simulink model "passive_balance"  (R2023b)
settings: Solver=VariableStepAuto  StartTime=0.0  StopTime=inf  RelTol=1e-3
undefined symbols (not defined in the file): Ion, LF, Lithium
libraries: instrumentseriallib x9, spsSeriesRLCBranchLib x4, spsBatteryLib x3, spsIGBTLib x3, etargetslib x3, spsIdealSwitchLib x2, spsDCVoltageSourceLib x1, spspowerguiLib x1
settings Model: Creator=ASUS  LastModifiedBy=Bramantio

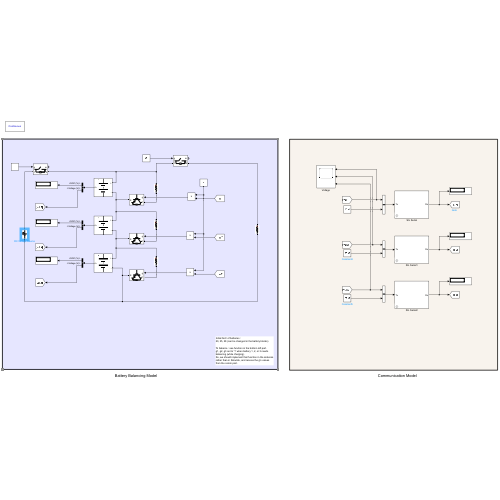
[thumbnail: Simulink's stored preview of the top-level diagram]
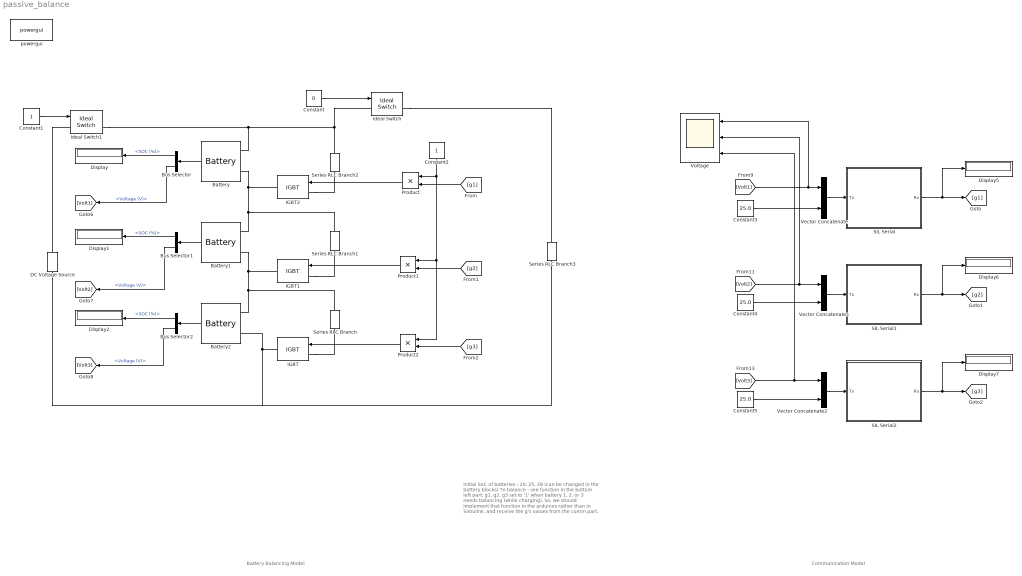
== system passive_balance ==
  note: Initial SoC of batteries :
      | 20, 25, 28 (can be changed in the battery blocks)
      |
      | To balance : see function in the bottom left part.
      | g1, g2, g3 set to '1' when battery 1, 2, or 3 needs
      | balancing (while charging).
      | So, we should implement that function in the arduinos
      | rather than in Simulink, and receive the g's values
      | from the comm part.
  note: Battery Balancing Model
  note: Communication Model
  Battery : spsBatteryLib/Battery  BatType=Lithium-Ion  ShowTempParam=off  ThermalPreset=no  ShowAgeParam=off  NomV=3.2  NomQ=180  SOC=20  Batt_Tr=30  PresetModel=on  MaxQ=180  MinV=2.4  FullV=3.7248  Dis_rate=78.2609  R=0.00017778  Normal_OP=162.7826  expZone="[3.4572      8.8435]"  current=[6.5 13 32.5]  Units=Time  Tci=20  NomT=20  T2=-30  MaxQ2=4.8  FullV2=7.1  Normal_OP2=5.655  expZone2="[6.58           1]"  Rca=0.6  ti=2000  Dp=0  Neq0=0  Tsim=1e6  Ta1=25  Qeol=5.4*0.9  Reol=0.013333*1.2  Char_age=[2.3478, 3]  Dis_age=[2.3478, 10]  N1=1500  N2=10500  N3=1000  N4=1400  Ta2=45  N5=950
  Battery1 : spsBatteryLib/Battery  BatType=Lithium-Ion  ShowTempParam=off  ThermalPreset=no  ShowAgeParam=off  NomV=3.2  NomQ=180  SOC=25  Batt_Tr=30  PresetModel=on  MaxQ=180  MinV=2.4  FullV=3.7248  Dis_rate=78.2609  R=0.00017778  Normal_OP=162.7826  expZone="[3.4572      8.8435]"  current=[6.5 13 32.5]  Units=Time  Tci=20  NomT=20  T2=-30  MaxQ2=4.8  FullV2=7.1  Normal_OP2=5.655  expZone2="[6.58           1]"  Rca=0.6  ti=2000  Dp=0  Neq0=0  Tsim=1e6  Ta1=25  Qeol=5.4*0.9  Reol=0.013333*1.2  Char_age=[2.3478, 3]  Dis_age=[2.3478, 10]  N1=1500  N2=10500  N3=1000  N4=1400  Ta2=45  N5=950
  Battery2 : spsBatteryLib/Battery  BatType=Lithium-Ion  ShowTempParam=off  ThermalPreset=no  ShowAgeParam=off  NomV=3.2  NomQ=180  SOC=28  Batt_Tr=30  PresetModel=on  MaxQ=180  MinV=2.4  FullV=3.7248  Dis_rate=78.2609  R=0.00017778  Normal_OP=162.7826  expZone="[3.4572      8.8435]"  current=[6.5 13 32.5]  Units=Time  Tci=20  NomT=20  T2=-30  MaxQ2=4.8  FullV2=7.1  Normal_OP2=5.655  expZone2="[6.58           1]"  Rca=0.6  ti=2000  Dp=0  Neq0=0  Tsim=1e6  Ta1=25  Qeol=5.4*0.9  Reol=0.013333*1.2  Char_age=[2.3478, 3]  Dis_age=[2.3478, 10]  N1=1500  N2=10500  N3=1000  N4=1400  Ta2=45  N5=950
  Bus Selector : BusSelector  OutputSignals=SOC (%),Voltage (V)
  Bus Selector1 : BusSelector  OutputSignals=SOC (%),Voltage (V)
  Bus Selector2 : BusSelector  OutputSignals=SOC (%),Voltage (V)
  Constant : Constant  Value=0
  Constant1 : Constant
  Constant2 : Constant
  Constant3 : Constant  Value=25.0
  Constant4 : Constant  Value=25.0
  Constant5 : Constant  Value=25.0
  DC Voltage Source : spsDCVoltageSourceLib/DC Voltage Source  Amplitude=10  Measurements=None
  Display{,1..2,5..7} (6 alike) : Display
  IGBT : spsIGBTLib/IGBT  Ron=0.001  Lon=0  Vf=1  Tf=1e-6  Tt=2e-6  IC=0  Rs=1e5  Cs=inf  Measurements=off
  IGBT1 : spsIGBTLib/IGBT  Ron=0.001  Lon=0  Vf=1  Tf=1e-6  Tt=2e-6  IC=0  Rs=1e5  Cs=inf  Measurements=off
  IGBT2 : spsIGBTLib/IGBT  Ron=0.001  Lon=0  Vf=1  Tf=1e-6  Tt=2e-6  IC=0  Rs=1e5  Cs=inf  Measurements=off
  Ideal Switch : spsIdealSwitchLib/Ideal Switch  Ron=0.001  Lon=0  IC=0  Rs=1e5  Cs=inf  Measurements=on
  Ideal Switch1 : spsIdealSwitchLib/Ideal Switch  Ron=0.001  Lon=0  IC=0  Rs=1e5  Cs=inf  Measurements=on
  Product : Product
  Product1 : Product
  Product2 : Product
  SIL Serial : Subsystem  mask{comport=COM3, data_size=1, sample_time=0.5, baud_rate=115200}
      mask prompts: comport "Serial Port (ex. "COM3")"; data_size "Data Size"; sample_time "Sample Time"; baud_rate "Baud Rate"
  SIL Serial1 : Subsystem  mask{comport=COM7, data_size=1, sample_time=0.5, baud_rate=115200}
      mask prompts: comport "Serial Port (ex. "COM3")"; data_size "Data Size"; sample_time "Sample Time"; baud_rate "Baud Rate"
  SIL Serial2 : Subsystem  mask{comport=COM8, data_size=1, sample_time=0.5, baud_rate=115200}
      mask prompts: comport "Serial Port (ex. "COM3")"; data_size "Data Size"; sample_time "Sample Time"; baud_rate "Baud Rate"
  Series RLC Branch{,1..3} (4 alike) : spsSeriesRLCBranchLib/Series RLC Branch  LConnTagsString=__new0  RConnTagsString=__new0  BranchType=R  Resistance=1  Inductance=1e-3  SetiL0=off  InitialCurrent=0  Capacitance=1e-6  Setx0=off  InitialVoltage=0  Measurements=None
  Vector Concatenate : Concatenate
  Vector Concatenate1 : Concatenate
  Vector Concatenate2 : Concatenate
  Voltage : Scope  NumInputPorts=3
  powergui : spspowerguiLib/powergui  Priority=1  SimulationMode=Continuous  SampleTime=50e-6  frequency=60  Iterations=50  frequencyindice=0  Pbase=100e6  ErrMax=1e-4  UnitsV=kV  UnitsW=MW  buscounter=0  FunctionMessages=off  echomessages=off  EnableUseOfTLC=off  CurrentSourceSwitches=off  DisableSnubberDevices=off  DisableRonSwitches=off  DisableVfSwitches=off  DisplayEquations=off  AutomaticDiscreteSolvers=off  SolverType=Tustin/Backward Euler (TBE)  Interpol=off  ExternalGateDelay=off  methode=off  Ts=100  x0status=blocks  SPID=on  SwTol=0  HookPort=off  NonlinearTolerance=1e-4  nMaxIteration=100  ContinueOnMaxIteration=off  RestoreLinks=warning  ResistiveCurrentMeasurement=off  Frange=[0:2:500]  Ylog=off  Xlog=on  ShowGrid=off  save=off  variable=ZData  structure=0  ZoomFFT=off  StartTime=0.0  cycles=1  DisplayStyle=1  fundamental=60  FreqAxis=off  MaxFrequency=1000  frequencyindicesteady=1  RmsSteady=1  display=off
  wires:
  Constant/1 -> Ideal Switch/1
  Constant1/1 -> Ideal Switch1/1
  Battery/1 -> Bus Selector/1
  Battery1/1 -> Bus Selector1/1
  Battery2/1 -> Bus Selector2/1
  Bus Selector/1 -> Display/1  "<SOC (%)>"
  Bus Selector1/1 -> Display1/1  "<SOC (%)>"
  Bus Selector2/1 -> Display2/1  "<SOC (%)>"
  Constant2/1 -> Product2/1, Product1/1, Product/1
  Product/1 -> IGBT2/1
  Product1/1 -> IGBT1/1
  Product2/1 -> IGBT/1
  [g1] -> Product/2
  [g2] -> Product1/2
  [g3] -> Product2/2
  Vector Concatenate2/1 -> SIL Serial2/1(Tx)
  Vector Concatenate1/1 -> SIL Serial1/1(Tx)
  Vector Concatenate/1 -> SIL Serial/1(Tx)
  [Volt1] -> Voltage/1, Vector Concatenate/1
  Bus Selector/2 -> [Volt1]  "<Voltage (V)>"
  Bus Selector1/2 -> [Volt2]  "<Voltage (V)>"
  [Volt2] -> Voltage/2, Vector Concatenate1/1
  Bus Selector2/2 -> [Volt3]  "<Voltage (V)>"
  [Volt3] -> Voltage/3, Vector Concatenate2/1
  SIL Serial/1(Rx) -> Display5/1, [g1]
  SIL Serial1/1(Rx) -> Display6/1, [g2]
  SIL Serial2/1(Rx) -> Display7/1, [g3]
  Constant3/1 -> Vector Concatenate/2
  Constant4/1 -> Vector Concatenate1/2
  Constant5/1 -> Vector Concatenate2/2
  connections:
  Battery/LConn2 -- IGBT2/RConn1 -- Series RLC Branch1/LConn1 -- Battery1/LConn1
  Battery1/LConn2 -- IGBT1/RConn1 -- Series RLC Branch/LConn1 -- Battery2/LConn1
  IGBT/RConn1 -- Battery2/LConn2 -- Series RLC Branch3/RConn1 -- DC Voltage Source/LConn1
  IGBT/LConn1 -- Series RLC Branch/RConn1
  IGBT1/LConn1 -- Series RLC Branch1/RConn1
  IGBT2/LConn1 -- Series RLC Branch2/RConn1
  Series RLC Branch2/LConn1 -- Ideal Switch/LConn1 -- Battery/LConn1 -- Ideal Switch1/RConn1
  DC Voltage Source/RConn1 -- Ideal Switch1/LConn1
  Ideal Switch/RConn1 -- Series RLC Branch3/LConn1

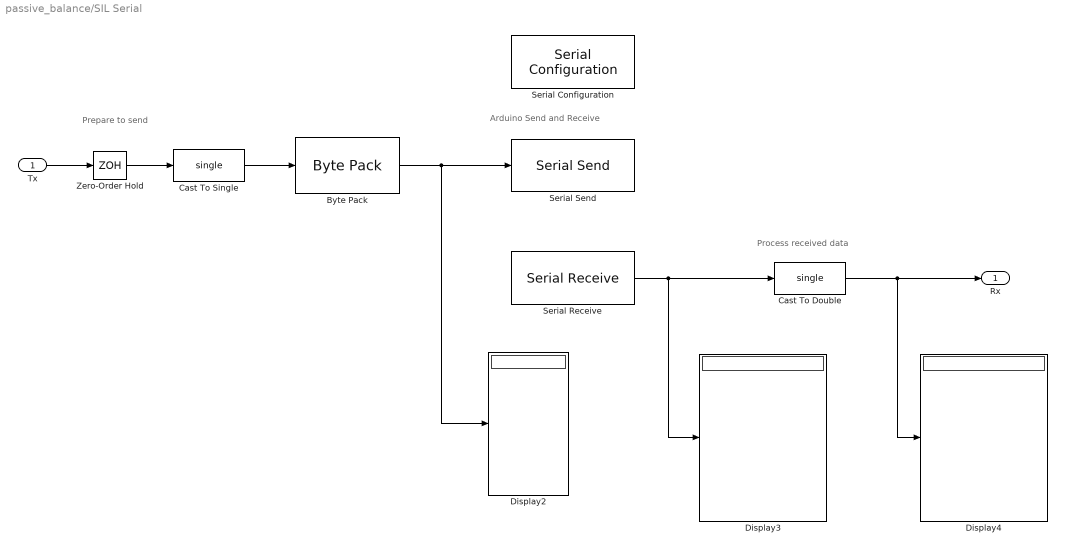
== system passive_balance/SIL Serial ==
  note: Prepare to send
  note: Arduino Send and Receive
  note: Process received data
  Tx : Inport
  Byte Pack : etargetslib/Byte Pack  datatypes={'single'}  byteAlign=4
  Cast To Double : DataTypeConversion  OutDataTypeStr=single  SaturateOnIntegerOverflow=off  RndMeth=Floor
  Cast To Single : DataTypeConversion  OutDataTypeStr=single  SaturateOnIntegerOverflow=off  RndMeth=Floor
  Display2 : Display
      settings: Format=hex (Stored Integer)
  Display3 : Display
  Display4 : Display
  Serial Configuration : instrumentseriallib/Serial Configuration  Priority=-200000  PortSel=comport  Port=comport  ComPort=comport  BaudRate=baud_rate  DataBits=8  Parity=none  StopBits=1  ByteOrder=little-endian  FlowControl=none  Timeout=10  SimulateUsing=Interpreted execution  BlockInModel=on  aMode=1
  Serial Receive : instrumentseriallib/Serial Receive  Priority=1  PortSel=comport  Port=comport  ComPort=comport  DataType=uint32  SaveDataType=uint8  ToggleHeader=on  Header=[ 65 ]  ToggleTerminator=on  Terminator=LF ('\n')  CustomTerminator=[]  InputFormat=Column major  ToggleDataSize=on  DataSize=[1 data_size]  EnableBlockingMode=on  ActionDataUnavailable=Output last received value  ActionWhenDataUnavailable=Output last received value  CustomValue=0  SampleTime=sample_time  SimulateUsing=Interpreted execution  BlockInModel=on  aMode=1
  Serial Send : instrumentseriallib/Serial Send  Priority=1  PortSel=comport  Port=comport  ComPort=comport  Header=[]  Terminator=LF ('\n')  CustomTerminator=[]  EnableBlockingMode=on  SimulateUsing=Interpreted execution  BlockInModel=on  aMode=1
  Zero-Order Hold : ZeroOrderHold  SampleTime=sample_time
  Rx : Outport
  wires:
  Tx/1 -> Zero-Order Hold/1
  Serial Receive/1 -> Display3/1, Cast To Double/1
  Zero-Order Hold/1 -> Cast To Single/1
  Byte Pack/1 -> Display2/1, Serial Send/1
  Cast To Double/1 -> Display4/1, Rx/1
  Cast To Single/1 -> Byte Pack/1

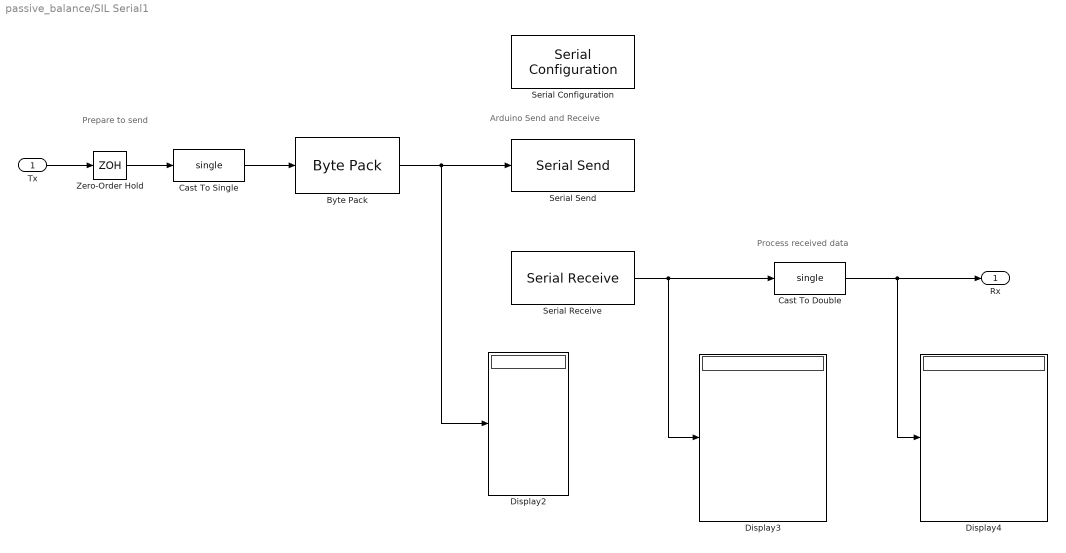
== system passive_balance/SIL Serial1 ==
  note: Prepare to send
  note: Arduino Send and Receive
  note: Process received data
  Tx : Inport
  Byte Pack : etargetslib/Byte Pack  datatypes={'single'}  byteAlign=4
  Cast To Double : DataTypeConversion  OutDataTypeStr=single  SaturateOnIntegerOverflow=off  RndMeth=Floor
  Cast To Single : DataTypeConversion  OutDataTypeStr=single  SaturateOnIntegerOverflow=off  RndMeth=Floor
  Display2 : Display
      settings: Format=hex (Stored Integer)
  Display3 : Display
  Display4 : Display
  Serial Configuration : instrumentseriallib/Serial Configuration  Priority=-200000  PortSel=comport  Port=comport  ComPort=comport  BaudRate=baud_rate  DataBits=8  Parity=none  StopBits=1  ByteOrder=little-endian  FlowControl=none  Timeout=10  SimulateUsing=Interpreted execution  BlockInModel=on  aMode=1
  Serial Receive : instrumentseriallib/Serial Receive  Priority=1  PortSel=comport  Port=comport  ComPort=comport  DataType=uint32  SaveDataType=uint8  ToggleHeader=on  Header=[ 65 ]  ToggleTerminator=on  Terminator=LF ('\n')  CustomTerminator=[]  InputFormat=Column major  ToggleDataSize=on  DataSize=[1 data_size]  EnableBlockingMode=on  ActionDataUnavailable=Output last received value  ActionWhenDataUnavailable=Output last received value  CustomValue=0  SampleTime=sample_time  SimulateUsing=Interpreted execution  BlockInModel=on  aMode=1
  Serial Send : instrumentseriallib/Serial Send  Priority=1  PortSel=comport  Port=comport  ComPort=comport  Header=[]  Terminator=LF ('\n')  CustomTerminator=[]  EnableBlockingMode=on  SimulateUsing=Interpreted execution  BlockInModel=on  aMode=1
  Zero-Order Hold : ZeroOrderHold  SampleTime=sample_time
  Rx : Outport
  wires:
  Tx/1 -> Zero-Order Hold/1
  Serial Receive/1 -> Display3/1, Cast To Double/1
  Zero-Order Hold/1 -> Cast To Single/1
  Byte Pack/1 -> Display2/1, Serial Send/1
  Cast To Double/1 -> Display4/1, Rx/1
  Cast To Single/1 -> Byte Pack/1

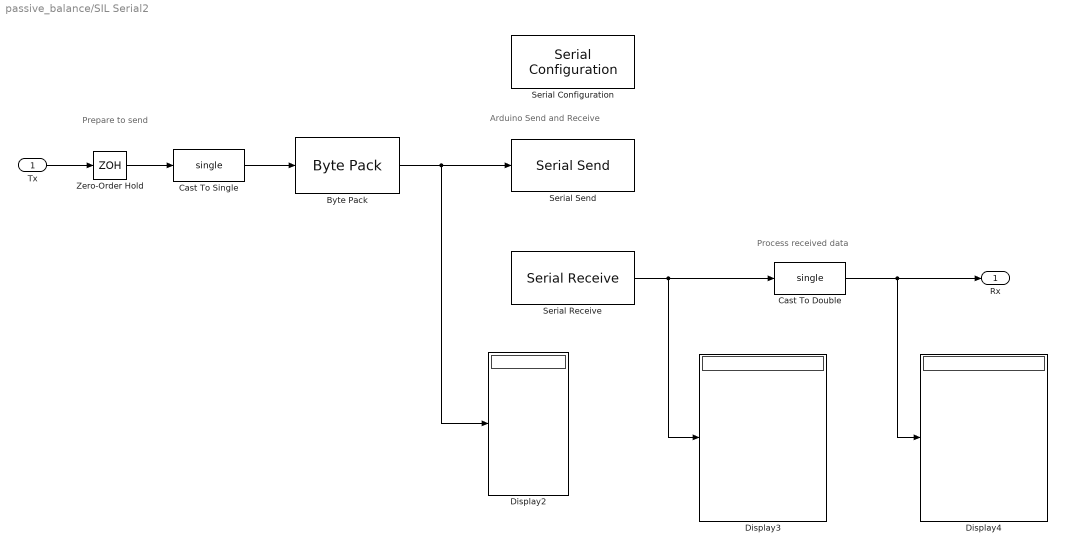
== system passive_balance/SIL Serial2 ==
  note: Prepare to send
  note: Arduino Send and Receive
  note: Process received data
  Tx : Inport
  Byte Pack : etargetslib/Byte Pack  datatypes={'single'}  byteAlign=4
  Cast To Double : DataTypeConversion  OutDataTypeStr=single  SaturateOnIntegerOverflow=off  RndMeth=Floor
  Cast To Single : DataTypeConversion  OutDataTypeStr=single  SaturateOnIntegerOverflow=off  RndMeth=Floor
  Display2 : Display
      settings: Format=hex (Stored Integer)
  Display3 : Display
  Display4 : Display
  Serial Configuration : instrumentseriallib/Serial Configuration  Priority=-200000  PortSel=comport  Port=comport  ComPort=comport  BaudRate=baud_rate  DataBits=8  Parity=none  StopBits=1  ByteOrder=little-endian  FlowControl=none  Timeout=10  SimulateUsing=Interpreted execution  BlockInModel=on  aMode=1
  Serial Receive : instrumentseriallib/Serial Receive  Priority=1  PortSel=comport  Port=comport  ComPort=comport  DataType=uint32  SaveDataType=uint8  ToggleHeader=on  Header=[ 65 ]  ToggleTerminator=on  Terminator=LF ('\n')  CustomTerminator=[]  InputFormat=Column major  ToggleDataSize=on  DataSize=[1 data_size]  EnableBlockingMode=on  ActionDataUnavailable=Output last received value  ActionWhenDataUnavailable=Output last received value  CustomValue=0  SampleTime=sample_time  SimulateUsing=Interpreted execution  BlockInModel=on  aMode=1
  Serial Send : instrumentseriallib/Serial Send  Priority=1  PortSel=comport  Port=comport  ComPort=comport  Header=[]  Terminator=LF ('\n')  CustomTerminator=[]  EnableBlockingMode=on  SimulateUsing=Interpreted execution  BlockInModel=on  aMode=1
  Zero-Order Hold : ZeroOrderHold  SampleTime=sample_time
  Rx : Outport
  wires:
  Tx/1 -> Zero-Order Hold/1
  Serial Receive/1 -> Display3/1, Cast To Double/1
  Zero-Order Hold/1 -> Cast To Single/1
  Byte Pack/1 -> Display2/1, Serial Send/1
  Cast To Double/1 -> Display4/1, Rx/1
  Cast To Single/1 -> Byte Pack/1
